simulink model "SF018A_EotProtn"  (R2013b)
settings: Solver=FixedStepDiscrete  SolverMode=SingleTasking  StartTime=0.0  StopTime=0.002  FixedStep=.002  RelTol=1e-3
undefined symbols (not defined in the file): ALLSPDDAMPG_CNT_U08, ALLSPDGAIN_CNT_U08, ARCHGLBPRM_2MILLISEC_SEC_F32, DISTLPFILFRQ_HZ_F32, EOTDAMPGLOLIM_MOTNWTMTR_F32, EOTGAINHILIM_ULS_F32, EotProtnActvRegnBypMaxThd, EotProtnDampgSlew, EotProtnDampgVehSpdTbl, EotProtnDeltaTqThd, EotProtnDftPosn, EotProtnEntrGainVehSpdTbl, EotProtnEntrGainX, EotProtnEntrStLpFilFrq, EotProtnExitDampgY, EotProtnExitStLpFilFrq, EotProtnHwAgGain, EotProtnHwAgMax, EotProtnHwAgMin, EotProtnHwDegDampgX, EotProtnMotSpdIncptSca, EotProtnMotSpdIncptX, EotProtnMotSpdIncptY, EotProtnMotVelGain, EotProtnNormDampgY, EotProtnPosnRampStep, EotProtnRackTrvlLimrAuthyThd, EotProtnRackTrvlLimrAuthyThdLimd, EotProtnRackTrvlLimrEna, EotProtnRackTrvlLimrRng, EotProtnRackTrvlLimrRngLimd, EotProtnRackTrvlLimrVehSpdThd, EotProtnRunEotVelImpctAndSoftEndStop, EotProtnSoftEndStopAuthyThd, EotProtnSoftEndStopEna, EotProtnSoftEndStopVehSpdThd, FIRSTPTDAMPG_CNT_U08, LASTPTGAIN_CNT_U08, SOFTENDSTOPSTDI_CNT_U08, SOFTENDSTOPSTENTR_CNT_U08, SOFTENDSTOPSTEXIT_CNT_U08, SOFTENDSTOPSTNORM_CNT_U08, SYSGLBPRM_MOTTQCMDHILIM_MOTNWTMTR_F32, ZEROMOTTQCMD_MOTNWTMTR_F32
libraries: NxtrAbslt x16, FloatToFixd x14, FixdToFloat x6, Fil x5, NxtrLim x5, simulink x4, NxtrMax x4, LnrIntrpnDyn x3, NxtrSign x2, BilnrIntrpnMplXDyn x2, BilnrIntrpnMplX x1, LnrIntrpn x1
(part 1 of 5)
settings Model: Creator=BZHF94  LastModifiedBy=HZQ8V7
settings DataIOCC: LimitDataPoints=off  SaveFormat=Structure  ReturnWorkspaceOutputs=on
settings OptimizationCC: BlockReduction=off  InlineParams=on  ZeroExternalMemoryAtStartup=off  ZeroInternalMemoryAtStartup=off  OptimizeModelRefInitCode=on  LifeSpan=1
settings DebuggingCC: SignalInfNanChecking=error  SignalRangeChecking=warning  UnderspecifiedInitializationDetection=Simplified  SolverPrmCheckMsg=error  InheritedTsInSrcMsg=error  DiscreteInheritContinuousMsg=error  MultiTaskDSMMsg=none  SingleTaskRateTransMsg=error  TasksWithSamePriorityMsg=error  SigSpecEnsureSampleTimeMsg=error  CheckMatrixSingularityMsg=error  IntegerOverflowMsg=none  ParameterOverflowMsg=none  ParameterUnderflowMsg=error  ParameterPrecisionLossMsg=error  ParameterTunabilityLossMsg=error  FixptConstUnderflowMsg=warning  FixptConstOverflowMsg=warning  VectorMatrixConversionMsg=error  SignalLabelMismatchMsg=error  UnconnectedInputMsg=error  UnconnectedOutputMsg=error  UnconnectedLineMsg=error  SFcnCompatibilityMsg=error  UniqueDataStoreMsg=warning  BusObjectLabelMismatch=error  RootOutportRequireBusObject=error  AssertControl=DisableAll  ModelReferenceIOMsg=error  ModelReferenceVersionMismatchMessage=warning  ModelReferenceIOMismatchMessage=error  ModelReferenceCSMismatchMessage=warning  ModelReferenceDataLoggingMessage=error  StateNameClashWarn=warning  StrictBusMsg=ErrorOnBusTreatedAsVector  NonBusSignalsTreatedAsBus=error  SFUnexpectedBacktrackingDiag=error  SFInvalidInputDataAccessInChartInitDiag=error  SFNoUnconditionalDefaultTransitionDiag=error  SFTransitionOutsideNaturalParentDiag=error  SFUnconditionalTransitionShadowingDiag=error  SFUndirectedBroadcastEventsDiag=error
settings ModelReferenceCC: ModelReferenceNumInstancesAllowed=Single
settings RTWCC: SystemTargetFile=autosar.tlc  GenCodeOnly=on  TemplateMakefile=ert_default_tmf  Description=AUTOSAR  GenerateReport=on  ProcessScript=autosar_make_rtw_hook  LaunchReport=on
settings CodeAppCC: GenerateComments=off  IgnoreCustomStorageClasses=off  CustomSymbolStrType=$N$R$M  CustomSymbolStrBlkIO=$N$M  SimulinkBlockComments=off
settings STFCustomTargetCC: ParMdlRefBuildCompliant=on  CompOptLevelCompliant=on  IncludeMdlTerminateFcn=off  CombineOutputUpdateFcns=on  SuppressErrorStatus=on  ERTFirstTimeCompliant=on  ERTCustomFileBanners=on  SupportNonFinite=off  SupportComplex=off  SupportContinuousTime=off  SupportNonInlinedSFcns=off  MATLABClassNameForMDSCustomization=Simulink.SoftwareTarget.ERTCustomization  AutosarCompliant=on  GRTInterface=off  SystemTargetFile=autosar.tlc
settings ERTTargetCC: CodeReplacementLibrary=ANSI_C  ConcurrentExecutionCompliant=off  IncludeMdlTerminateFcn=off  SuppressErrorStatus=on  SupportNonFinite=off  SupportComplex=off  ModelStepFunctionPrototypeControlCompliant=off  CPPClassGenCompliant=off  AutosarCompliant=on  InlinedParameterPlacement=NonHierarchical  ERTCustomFileTemplate=example_file_process.tlc  EnableUserReplacementTypes=on

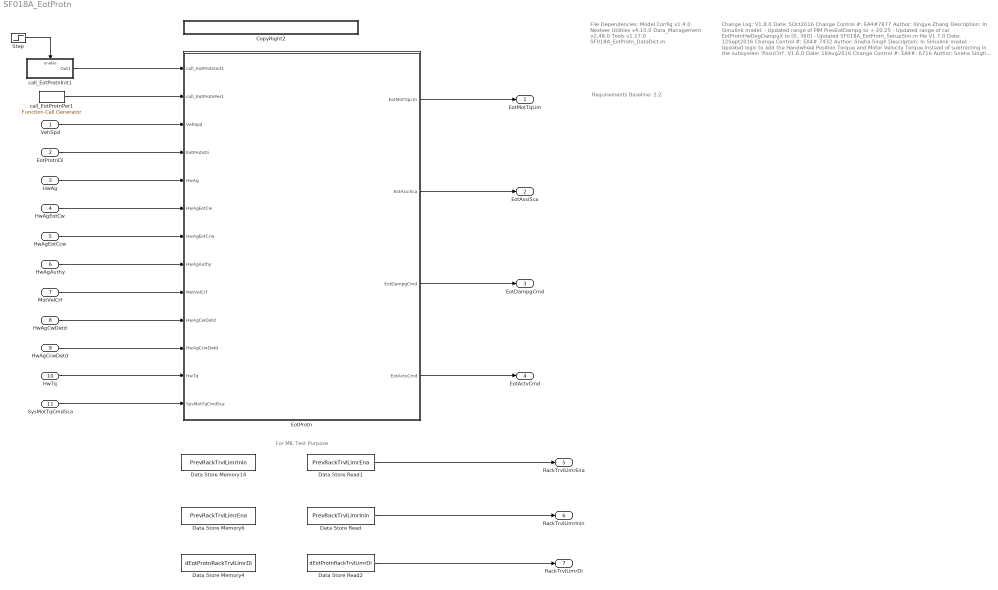
== system SF018A_EotProtn ==
  note: For MIL Test Purpose
  note: File Dependencies:
      |
      | Model Config v1.4.0
      | Nexteer Utilities v4.10.0
      | Data_Management v2.48.0
      | Tools v1.17.0
      | SF018A_EotProtn_DataDict.m
  note: Requirements Baseline: 2.2
  note: Change Log:
      |
      | V1.8.0
      | Date: 5Oct2016
      | Change Control #: EA4#7877
      | Author: Xingye Zhang
      | Description:
      | In Simulink model:
      | - Updated range of PIM PrevEotDampg to +-20.25
      | - Updated range of cal EotProtnHwDegDampgX to [0, 360]
      | - Updated  SF018A_EotProtn_SetupSim.m file
      |
      | V1.7.0
      | Date: 12Sept2016
      | Change Control #: EA4# 7432
      | Author: Sneha Singh
      | Description:
      | In Simulink model:
      | - Updated logic to add the Handwheel Position Torque and Motor Velocity
      | Torque instead of subtracting in the subsystem 'PosnCtrl'.
      |
      | V1.6.0
      | Date: 18Aug2016
      | Change Control #: EA4#: 6716
      | Author: Sneha Singh
      | Description:
      | In DataDictionary:
      | - Updated the filter gain and state variable range.
      | - Updated graphlink for 'EotProtnEntrGainY'.
      | In Simulink model:
      | - Initial values for filter data store blocks updated.
      | - Execution order of 'PrevSoftEndStopSt' updated to read before write.
      | - Deleted AND and NOT blocks from the subsystem 'RackTrvlLimrInin'.
      |
      | V1.5.0
      | Date: 12Jun2016
      | Change Control #: EA4#: 6120
      | Author: Harsh Karve
      | Description
      | In DataDictionary: Added EotProtnRackTrvlLimrAuthyThdLimd
      | 	and EotProtnRackTrvlLimrRngLimd
      | In Simulink model: Added logic to select between
      | 	EotProtnRackTrvlLimrRngLimd and EotProtnRackTrvlLimrRng
      | 	based on EotProtnRackTrvlLimrAuthyThd
      | 	and EotProtnRackTrvlLimrAuthyThdLimd
      |
      | V1.4.0
      | Date: 12Jan2016
      | Change Control #: EA4#3273
      | Author: Sudeep Shankar
      | Description:
      | In DataDictionary, EotProtnRackTrvlLimrEna.EngVal default changed
      | from
      | 1 to 0 to maintain consistency with SF-11
      |
      | V1.3.0
      | Date: 05Oct2015
      | Change Control #: EA4#1019
      | Author: Fei Yuan
      | Description:
      | - Minor values changes on the calibrations:
      |       EotProtnDampgVehSpdTbl
      | 	 EotProtnDftPosn
      | 	 EotProtnEntrGainY
      | 	 EotProtnHwDegDampgX
      | 	 EotProtnMotSpdIncptX
      | 	 EotProtnMotSpdIncptY
      | 	 EotProtnExitDampgY
      |  	 EotProtnNormDampgY
      |  	 EotProtnRackTrvlLimrRng
      |  	 EotProtnRackTrvlLimrVehSpdThd
      |  	 EotProtnSoftEndStopAuthyThd
      | - Unit changes from 'Uls' to 'Cnt' on the constants:
      | 	 ALLSPDDAMPG_CNT_U08
      | 	 ALLSPDGAIN_CNT_U08
      | 	 FIRSTPTDAMPG_CNT_U08
      | 	 LASTPTGAIN_CNT_U08
      |
      |
      | V1.2.0
      | Date: 01Oct2015
      | Change Control #: EA4#1019
      | Author: Fei Yuan
      | Description:
      | - EotAssiSca.WrittenIn is added.
      | - PrevHwTqLpFil is changed to HwTqLpFil.
      | - PrevEotAssiScaLpFil is changed to EotAssiScaLpFil.
      | - LASTROWGAIN_ULS_F32 is changed to LASTPTGAIN_ULS_U08.
      | - FIRSTROWDAMPG_ULS_F32 is changed to FIRSTPTDAMPG_ULS_U08.
      | - ALLCOLGAIN_ULS_F32 is changed to ALLSPDGAIN_ULS_U08.
      | - ALLCOLDAMPG_ULS_U08 is changed to ALLSPDDAMPG_ULS_U08.
      |
      |
      | V 1.1.0
      | Date: 28Sep2015
      | Change Control #: EA4#1019
      | Author: Fei Yuan
      | Description:
      | - Deleting unneeded imported calibration
      | in the Data Dictionary
      |
      |
      | V 1.0.0
      | Date: 15Sep2015
      | Change Control #: EA4#1019
      | Author: Fei Yuan
      | Description:
      | - Initial Release Based on EA3 V 1.0.0
  VehSpd : Inport  RequirementInfo={} %GIDa_f2493df3_3560_4e8c_9ac3_cc4ada172b3a
  EotProtnDi : Inport  RequirementInfo={} %GIDa_9947c430_a5d7_4588_95dd_03f461632271  Port=2
  HwAg : Inport  RequirementInfo={} %GIDa_2659bb7a_c59e_415b_8b99_460c1be3fe4a  Port=3
  HwAgEotCw : Inport  RequirementInfo={} %GIDa_b8d4db66_b9a1_483c_9e62_5724d2f818de  Port=4
  HwAgEotCcw : Inport  RequirementInfo={} %GIDa_ddb9e909_8804_448b_851e_077ef608e27a  Port=5
  HwAgAuthy : Inport  RequirementInfo={} %GIDa_073559df_e8e0_40c2_83ff_8c97959cf4b7  Port=6
  MotVelCrf : Inport  RequirementInfo={} %GIDa_06a07364_6048_4403_8ccd_af20484cf926  Port=7
  HwAgCwDetd : Inport  RequirementInfo={} %GIDa_c86b3aa5_494e_4d5c_8b58_596cd01b1b79  Port=8
  HwAgCcwDetd : Inport  RequirementInfo={} %GIDa_6f73f07d_03be_4ab3_ac9e_f6331c6d0b68  Port=9
  HwTq : Inport  RequirementInfo={} %GIDa_3422e606_a4dc_43df_b15d_a957c57f1483  Port=10
  SysMotTqCmdSca : Inport  RequirementInfo={} %GIDa_5f2ee495_d7fd_4bfd_8356_7328f9a76091  Port=11
  CopyRight2 : Subsystem  Description=|  mask(Copyright Information){none=on}
      | Copyright info block.                                               
      |                                                                     
      | Place copyright information at the top of every subsystem in design.
      mask prompts: none "No parameters"
      mask help: Place copyright information at the top of every subsystem in design.
      mask Display:
      | NxtrConf = 'Nexteer Confidential';
      | 
      | sys = bdroot; %handle for the current model ("system")
      | first = get_param(sys,'Created');
      | if(isempty(first))
      |     first = datestr(now,'yyyy');
      | else
      |     first = first(end-3:end);  %year is last four digits
      | end
      | 
      | last = get_param(sys,'LastModifiedDate');
      | if isempty(last)
      |     last = datestr(now,'yyyy');
      | else
      |     last = last(end-3:end);
      | end
      | 
      | if strcmp(first,last)
      |     fprintf('%s -- Copyright %s Nexteer',NxtrConf,first)
      | else
      |     fprintf('%s -- %s%s- %s Nexteer',NxtrConf,char(169),first,last)
      | end
  Data Store Memory14 : DataStoreMemory  DataStoreName=PrevRackTrvlLimrInin  StateMustResolveToSignalObject=on
  Data Store Memory4 : DataStoreMemory  DataStoreName=dEotProtnRackTrvlLimrDi  StateMustResolveToSignalObject=on
  Data Store Memory6 : DataStoreMemory  DataStoreName=PrevRackTrvlLimrEna  StateMustResolveToSignalObject=on
  Data Store Read : DataStoreRead  DataStoreName=PrevRackTrvlLimrInin  SampleTime=0.002
  Data Store Read1 : DataStoreRead  DataStoreName=PrevRackTrvlLimrEna  SampleTime=0.002
  Data Store Read2 : DataStoreRead  DataStoreName=dEotProtnRackTrvlLimrDi  SampleTime=0.002
  EotProtn : Subsystem
  Step : Step  Time=.001  Before=1  After=0  SampleTime=0
  call_EotProtnInit1 : Subsystem  TreatAsAtomicUnit=on
  call_EotProtnPer1 : simulink/Ports & Subsystems/Function-Call Generator  RequirementInfo={} %GIDa_6f959799_a3aa_4853_a8c2_1b349d8a0077  sample_time=0.002  numberOfIterations=1
  EotMotTqLim : Outport
  EotAssiSca : Outport  Port=2
  EotDampgCmd : Outport  Port=3
  EotActvCmd : Outport  Port=4
  RackTrvlLimrEna : Outport  Port=5
  RackTrvlLimrInin : Outport  Port=6
  RackTrvlLimrDi : Outport  Port=7
  wires:
  EotProtn/1(EotMotTqLim) -> EotMotTqLim/1
  EotProtn/4(EotActvCmd) -> EotActvCmd/1
  EotProtn/3(EotDampgCmd) -> EotDampgCmd/1
  EotProtn/2(EotAssiSca) -> EotAssiSca/1
  Data Store Read/1 -> RackTrvlLimrInin/1
  Data Store Read1/1 -> RackTrvlLimrEna/1
  Data Store Read2/1 -> RackTrvlLimrDi/1
  Step/1 -> call_EotProtnInit1/Enable
  call_EotProtnPer1/1 -> EotProtn/2(call_EotProtnPer1)
  call_EotProtnInit1/1(Out1) -> EotProtn/1(call_EotProtnInit1)
  VehSpd/1 -> EotProtn/3(VehSpd)
  EotProtnDi/1 -> EotProtn/4(EotProtnDi)
  HwAg/1 -> EotProtn/5(HwAg)
  HwAgEotCw/1 -> EotProtn/6(HwAgEotCw)
  HwAgEotCcw/1 -> EotProtn/7(HwAgEotCcw)
  HwAgAuthy/1 -> EotProtn/8(HwAgAuthy)
  MotVelCrf/1 -> EotProtn/9(MotVelCrf)
  HwAgCwDetd/1 -> EotProtn/10(HwAgCwDetd)
  HwAgCcwDetd/1 -> EotProtn/11(HwAgCcwDetd)
  HwTq/1 -> EotProtn/12(HwTq)
  SysMotTqCmdSca/1 -> EotProtn/13(SysMotTqCmdSca)

== system SF018A_EotProtn/CopyRight2 ==

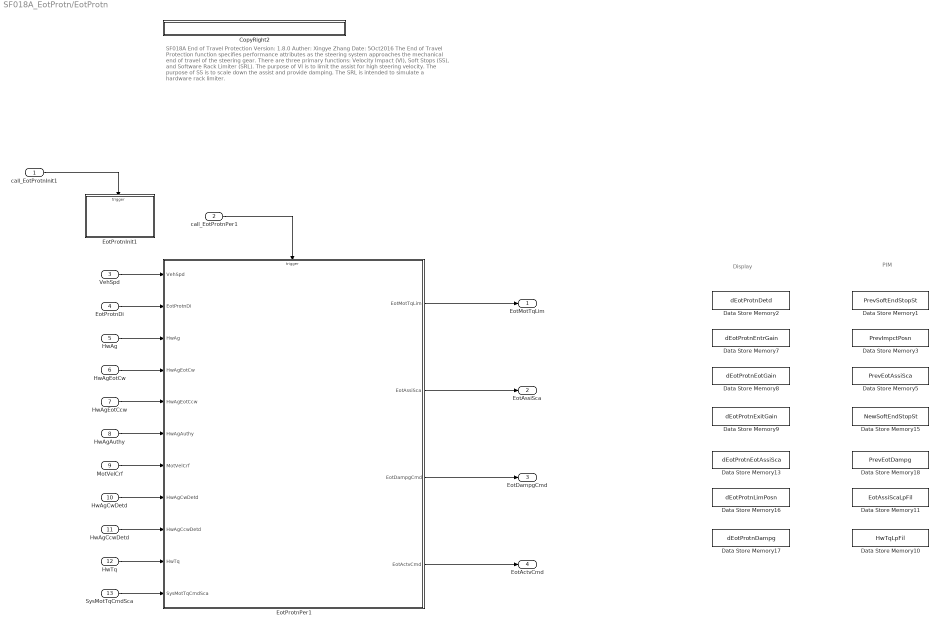
== system SF018A_EotProtn/EotProtn ==
  note: PIM
  note: Display
  note: SF018A End of Travel Protection
      | Version: 1.8.0  Auther: Xingye Zhang       Date: 5Oct2016
      |
      | The End of Travel Protection function specifies performance attributes as the steering system approaches the mechanical end of travel
      | of the steering gear. There are three primary functions: Velocity Impact (VI), Soft Stops (SS), and Software Rack Limiter (SRL).
      |
      | The purpose of VI is to limit the assist for high steering velocity. The purpose of SS is to scale down the assist and provide damping. The
      | SRL is intended to simulate a hardware rack limiter.
  call_EotProtnInit1 : Inport
  call_EotProtnPer1 : Inport  Port=2
  VehSpd : Inport  RequirementInfo={'linktype_rmi_doors' '0000ba56 (/E-STEER Core/SubSystem Specifications/Application Functions/SF018A End-of-Travel Actuator Management- EOT Impact and Soft Stops)' '#SF018A_39' 'true' 'REQ: SF018A_39' '' } %GIDa_a78556f8_403e_4502_952b_ada00a94acb5  Port=3
  EotProtnDi : Inport  RequirementInfo={'linktype_rmi_doors' '0000ba56 (/E-STEER Core/SubSystem Specifications/Application Functions/SF018A End-of-Travel Actuator Management- EOT Impact and Soft Stops)' '#SF018A_40' 'true' 'REQ: SF018A_40' '' } %GIDa_b64a771e_65c5_4ece_b91a_db7d931b086f  Port=4
  HwAg : Inport  RequirementInfo={'linktype_rmi_doors' '0000ba56 (/E-STEER Core/SubSystem Specifications/Application Functions/SF018A End-of-Travel Actuator Management- EOT Impact and Soft Stops)' '#SF018A_41' 'true' 'REQ: SF018A_41' '' } %GIDa_eecdc59f_15cc_4f2b_ad72_cb34d73e8cb8  Port=5
  HwAgEotCw : Inport  RequirementInfo={'linktype_rmi_doors' '0000ba56 (/E-STEER Core/SubSystem Specifications/Application Functions/SF018A End-of-Travel Actuator Management- EOT Impact and Soft Stops)' '#SF018A_81' 'true' 'REQ: SF018A_81' '' } %GIDa_23f8dc21_a30b_406d_bb74_847676667852  Port=6
  HwAgEotCcw : Inport  RequirementInfo={'linktype_rmi_doors' '0000ba56 (/E-STEER Core/SubSystem Specifications/Application Functions/SF018A End-of-Travel Actuator Management- EOT Impact and Soft Stops)' '#SF018A_82' 'true' 'REQ: SF018A_82' '' } %GIDa_6c945122_f602_4615_8a0d_9b6a5b36fdce  Port=7
  HwAgAuthy : Inport  RequirementInfo={'linktype_rmi_doors' '0000ba56 (/E-STEER Core/SubSystem Specifications/Application Functions/SF018A End-of-Travel Actuator Management- EOT Impact and Soft Stops)' '#SF018A_42' 'true' 'REQ: SF018A_42' '' } %GIDa_097a9b08_a5d5_46d9_827a_8d91469ca1ea  Port=8
  MotVelCrf : Inport  RequirementInfo={'linktype_rmi_doors' '0000ba56 (/E-STEER Core/SubSystem Specifications/Application Functions/SF018A End-of-Travel Actuator Management- EOT Impact and Soft Stops)' '#SF018A_38' 'true' 'REQ: SF018A_38' '' } %GIDa_1a8588a9_3d2e_48f3_a762_af26475c6c5c  Port=9
  HwAgCwDetd : Inport  RequirementInfo={'linktype_rmi_doors' '0000ba56 (/E-STEER Core/SubSystem Specifications/Application Functions/SF018A End-of-Travel Actuator Management- EOT Impact and Soft Stops)' '#SF018A_43' 'true' 'REQ: SF018A_43' '' } %GIDa_b5da2d0c_99ae_4332_b60f_c5663cccbdf6  Port=10
  HwAgCcwDetd : Inport  RequirementInfo={'linktype_rmi_doors' '0000ba56 (/E-STEER Core/SubSystem Specifications/Application Functions/SF018A End-of-Travel Actuator Management- EOT Impact and Soft Stops)' '#SF018A_80' 'true' 'REQ: SF018A_80' '' } %GIDa_337a4959_1d61_4717_9ff7_4d7f36a2ed66  Port=11
  HwTq : Inport  RequirementInfo={'linktype_rmi_doors' '0000ba56 (/E-STEER Core/SubSystem Specifications/Application Functions/SF018A End-of-Travel Actuator Management- EOT Impact and Soft Stops)' '#SF018A_18' 'true' 'REQ: SF018A_18' '' } %GIDa_c0387548_ba78_41a1_af32_a62cdacc5f34  Port=12
  SysMotTqCmdSca : Inport  RequirementInfo={'linktype_rmi_doors' '0000ba56 (/E-STEER Core/SubSystem Specifications/Application Functions/SF018A End-of-Travel Actuator Management- EOT Impact and Soft Stops)' '#SF018A_156' 'true' 'REQ: SF018A_156' '' } %GIDa_0ae76b0a_9341_4fdf_8ebd_214537950b15  Port=13
  CopyRight2 : Subsystem  Description=|  mask(Copyright Information){none=on}
      | Copyright info block.                                               
      |                                                                     
      | Place copyright information at the top of every subsystem in design.
      mask prompts: none "No parameters"
      mask help: Place copyright information at the top of every subsystem in design.
      mask Display:
      | NxtrConf = 'Nexteer Confidential';
      | 
      | sys = bdroot; %handle for the current model ("system")
      | first = get_param(sys,'Created');
      | if(isempty(first))
      |     first = datestr(now,'yyyy');
      | else
      |     first = first(end-3:end);  %year is last four digits
      | end
      | 
      | last = get_param(sys,'LastModifiedDate');
      | if isempty(last)
      |     last = datestr(now,'yyyy');
      | else
      |     last = last(end-3:end);
      | end
      | 
      | if strcmp(first,last)
      |     fprintf('%s -- Copyright %s Nexteer',NxtrConf,first)
      | else
      |     fprintf('%s -- %s%s- %s Nexteer',NxtrConf,char(169),first,last)
      | end
  Data Store Memory1 : DataStoreMemory  DataStoreName=PrevSoftEndStopSt  StateMustResolveToSignalObject=on
  Data Store Memory10 : DataStoreMemory  DataStoreName=HwTqLpFil  InitialValue=[]  OutDataTypeStr=Bus: FilLpRec1  StateMustResolveToSignalObject=on
  Data Store Memory11 : DataStoreMemory  DataStoreName=EotAssiScaLpFil  InitialValue=[]  OutDataTypeStr=Bus: FilLpRec1  StateMustResolveToSignalObject=on
  Data Store Memory13 : DataStoreMemory  DataStoreName=dEotProtnEotAssiSca  ReadBeforeWriteMsg=warning  WriteAfterWriteMsg=warning  WriteAfterReadMsg=warning  StateMustResolveToSignalObject=on
  Data Store Memory15 : DataStoreMemory  DataStoreName=NewSoftEndStopSt  StateMustResolveToSignalObject=on
  Data Store Memory16 : DataStoreMemory  DataStoreName=dEotProtnLimPosn  ReadBeforeWriteMsg=warning  WriteAfterWriteMsg=warning  WriteAfterReadMsg=warning  StateMustResolveToSignalObject=on
  Data Store Memory17 : DataStoreMemory  DataStoreName=dEotProtnDampg  ReadBeforeWriteMsg=warning  WriteAfterWriteMsg=warning  WriteAfterReadMsg=warning  StateMustResolveToSignalObject=on
  Data Store Memory18 : DataStoreMemory  DataStoreName=PrevEotDampg  StateMustResolveToSignalObject=on
  Data Store Memory2 : DataStoreMemory  DataStoreName=dEotProtnDetd  ReadBeforeWriteMsg=warning  WriteAfterWriteMsg=warning  WriteAfterReadMsg=warning  StateMustResolveToSignalObject=on
  Data Store Memory3 : DataStoreMemory  DataStoreName=PrevImpctPosn  StateMustResolveToSignalObject=on
  Data Store Memory5 : DataStoreMemory  DataStoreName=PrevEotAssiSca  StateMustResolveToSignalObject=on
  Data Store Memory7 : DataStoreMemory  DataStoreName=dEotProtnEntrGain  ReadBeforeWriteMsg=warning  WriteAfterWriteMsg=warning  WriteAfterReadMsg=warning  StateMustResolveToSignalObject=on
  Data Store Memory8 : DataStoreMemory  DataStoreName=dEotProtnEotGain  ReadBeforeWriteMsg=warning  WriteAfterWriteMsg=warning  WriteAfterReadMsg=warning  StateMustResolveToSignalObject=on
  Data Store Memory9 : DataStoreMemory  DataStoreName=dEotProtnExitGain  ReadBeforeWriteMsg=warning  WriteAfterWriteMsg=warning  WriteAfterReadMsg=warning  StateMustResolveToSignalObject=on
  EotProtnInit1 : Subsystem
  EotProtnPer1 : Subsystem
  EotMotTqLim : Outport  RequirementInfo={'linktype_rmi_doors' '0000ba56 (/E-STEER Core/SubSystem Specifications/Application Functions/SF018A End-of-Travel Actuator Management- EOT Impact and Soft Stops)' '#SF018A_20' 'true' 'REQ: SF018A_20' '' } %GIDa_69ec1092_67bc_4a3b_9f2e_0b0963ae28ca
  EotAssiSca : Outport  RequirementInfo={'linktype_rmi_doors' '0000ba56 (/E-STEER Core/SubSystem Specifications/Application Functions/SF018A End-of-Travel Actuator Management- EOT Impact and Soft Stops)' '#SF018A_44' 'true' 'REQ: SF018A_44' '' } %GIDa_1d9dfd8d_4c50_4570_b0ff_14c703a96e1d  Port=2
  EotDampgCmd : Outport  RequirementInfo={'linktype_rmi_doors' '0000ba56 (/E-STEER Core/SubSystem Specifications/Application Functions/SF018A End-of-Travel Actuator Management- EOT Impact and Soft Stops)' '#SF018A_45' 'true' 'REQ: SF018A_45' '' } %GIDa_758b54e5_2560_4187_be88_11d99f480d4d  Port=3
  EotActvCmd : Outport  RequirementInfo={'linktype_rmi_doors' '0000ba56 (/E-STEER Core/SubSystem Specifications/Application Functions/SF018A End-of-Travel Actuator Management- EOT Impact and Soft Stops)' '#SF018A_83' 'true' 'REQ: SF018A_83' '' } %GIDa_02248581_82c0_43b2_970c_42c45dcb5430  Port=4
  wires:
  SysMotTqCmdSca/1 -> EotProtnPer1/11(SysMotTqCmdSca)
  call_EotProtnInit1/1 -> EotProtnInit1/Trigger
  call_EotProtnPer1/1 -> EotProtnPer1/Trigger
  HwAg/1 -> EotProtnPer1/3(HwAg)
  HwAgCcwDetd/1 -> EotProtnPer1/9(HwAgCcwDetd)
  EotProtnPer1/3(EotDampgCmd) -> EotDampgCmd/1
  HwAgEotCcw/1 -> EotProtnPer1/5(HwAgEotCcw)
  VehSpd/1 -> EotProtnPer1/1(VehSpd)
  HwAgEotCw/1 -> EotProtnPer1/4(HwAgEotCw)
  EotProtnDi/1 -> EotProtnPer1/2(EotProtnDi)
  HwAgCwDetd/1 -> EotProtnPer1/8(HwAgCwDetd)
  EotProtnPer1/2(EotAssiSca) -> EotAssiSca/1
  HwTq/1 -> EotProtnPer1/10(HwTq)
  MotVelCrf/1 -> EotProtnPer1/7(MotVelCrf)
  EotProtnPer1/1(EotMotTqLim) -> EotMotTqLim/1
  EotProtnPer1/4(EotActvCmd) -> EotActvCmd/1
  HwAgAuthy/1 -> EotProtnPer1/6(HwAgAuthy)

== system SF018A_EotProtn/call_EotProtnInit1 ==
  Enable : EnablePort
  CopyRight2 : Subsystem  Description=|  mask(Copyright Information){none=on}
      | Copyright info block.                                               
      |                                                                     
      | Place copyright information at the top of every subsystem in design.
      mask prompts: none "No parameters"
      mask help: Place copyright information at the top of every subsystem in design.
      mask Display:
      | NxtrConf = 'Nexteer Confidential';
      | 
      | sys = bdroot; %handle for the current model ("system")
      | first = get_param(sys,'Created');
      | if(isempty(first))
      |     first = datestr(now,'yyyy');
      | else
      |     first = first(end-3:end);  %year is last four digits
      | end
      | 
      | last = get_param(sys,'LastModifiedDate');
      | if isempty(last)
      |     last = datestr(now,'yyyy');
      | else
      |     last = last(end-3:end);
      | end
      | 
      | if strcmp(first,last)
      |     fprintf('%s -- Copyright %s Nexteer',NxtrConf,first)
      | else
      |     fprintf('%s -- %s%s- %s Nexteer',NxtrConf,char(169),first,last)
      | end
  Function_Call_Generator : simulink/Ports & Subsystems/Function-Call Generator  sample_time=0  numberOfIterations=1
  Out1 : Outport
  wires:
  Function_Call_Generator/1 -> Out1/1

== system SF018A_EotProtn/EotProtn/CopyRight2 ==

== system SF018A_EotProtn/EotProtn/EotProtnInit1 ==
  function : TriggerPort  TriggerType=function-call
  CopyRight2 : Subsystem  Description=|  mask(Copyright Information){none=on}
      | Copyright info block.                                               
      |                                                                     
      | Place copyright information at the top of every subsystem in design.
      mask prompts: none "No parameters"
      mask help: Place copyright information at the top of every subsystem in design.
      mask Display:
      | NxtrConf = 'Nexteer Confidential';
      | 
      | sys = bdroot; %handle for the current model ("system")
      | first = get_param(sys,'Created');
      | if(isempty(first))
      |     first = datestr(now,'yyyy');
      | else
      |     first = first(end-3:end);  %year is last four digits
      | end
      | 
      | last = get_param(sys,'LastModifiedDate');
      | if isempty(last)
      |     last = datestr(now,'yyyy');
      | else
      |     last = last(end-3:end);
      | end
      | 
      | if strcmp(first,last)
      |     fprintf('%s -- Copyright %s Nexteer',NxtrConf,first)
      | else
      |     fprintf('%s -- %s%s- %s Nexteer',NxtrConf,char(169),first,last)
      | end
  EotAssiScaLpFil : Fil/FilLpInit  RequirementInfo={'linktype_rmi_doors' '0000ba56 (/E-STEER Core/SubSystem Specifications/Application Functions/SF018A End-of-Travel Actuator Management- EOT Impact and Soft Stops)' '#SF018A_111' 'true' 'REQ: SF018A_111' '' } %GIDa_a2f99997_2c39_4020_9932_83fabe8f4401  Ic=0  Ts=ARCHGLBPRM_2MILLISEC_SEC_F32  Freq=DISTLPFILFRQ_HZ_F32  StVar=EotAssiScaLpFil
  HwTqLpFil : Fil/FilLpInit  Ic=0  Ts=ARCHGLBPRM_2MILLISEC_SEC_F32  Freq=EotProtnHwTqLpFilFrq  StVar=HwTqLpFil

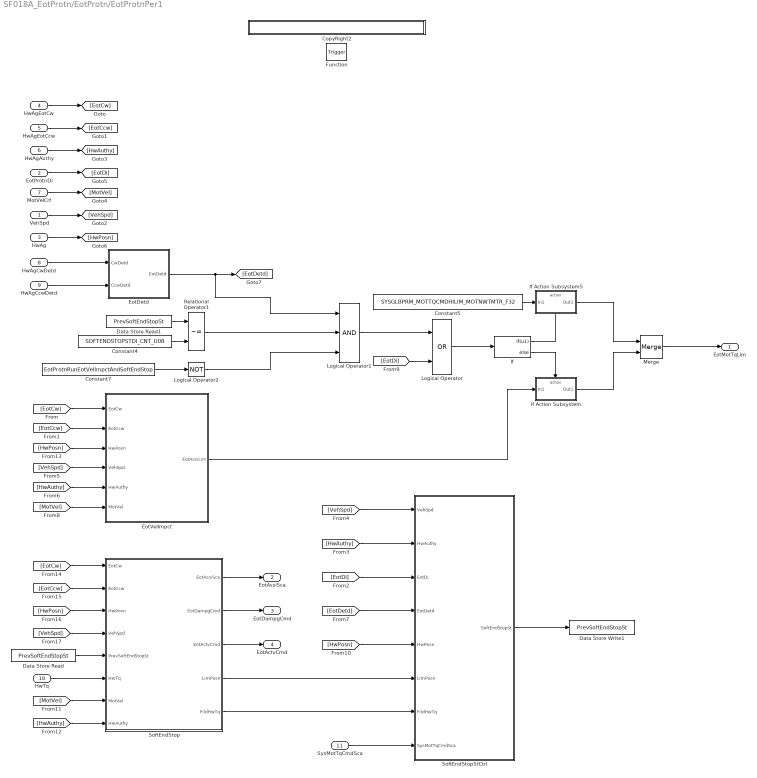
== system SF018A_EotProtn/EotProtn/EotProtnPer1 ==
  VehSpd : Inport
  EotProtnDi : Inport  Port=2
  HwAg : Inport  Port=3
  HwAgEotCw : Inport  Port=4
  HwAgEotCcw : Inport  Port=5
  HwAgAuthy : Inport  Port=6
  MotVelCrf : Inport  Port=7
  HwAgCwDetd : Inport  Port=8
  HwAgCcwDetd : Inport  Port=9
  HwTq : Inport  Port=10
  SysMotTqCmdSca : Inport  Port=11
  Function : TriggerPort  TriggerType=function-call  PortDimensions=1
  Constant4 : Constant  RequirementInfo={'linktype_rmi_doors' '0000ba56 (/E-STEER Core/SubSystem Specifications/Application Functions/SF018A End-of-Travel Actuator Management- EOT Impact and Soft Stops)' '#SF018A_101' 'true' 'REQ: SF018A_101' '' ; 'linktype_rmi_doors' '0000ba56 (/E-STEER Core/SubSystem Specifications/Application Functions/SF018A End-of-Travel Actuator Management- EOT Impact and Soft Stops)' '#SF018A_102' 'true' 'REQ: SF018A_102' '' } %GIDa_61ceba65_7d2a_487b_92a1_1928ed0fb012  Value=SOFTENDSTOPSTDI_CNT_U08
  Constant5 : Constant  RequirementInfo={'linktype_rmi_doors' '0000ba56 (/E-STEER Core/SubSystem Specifications/Application Functions/SF018A End-of-Travel Actuator Management- EOT Impact and Soft Stops)' '#SF018A_98' 'true' 'REQ: SF018A_98' '' } %GIDa_90b24707_b12d_4a90_a810_c09b59997368  Value=SYSGLBPRM_MOTTQCMDHILIM_MOTNWTMTR_F32
  Constant7 : Constant  RequirementInfo={'linktype_rmi_doors' '0000ba56 (/E-STEER Core/SubSystem Specifications/Application Functions/SF018A End-of-Travel Actuator Management- EOT Impact and Soft Stops)' '#SF018A_101' 'true' 'REQ: SF018A_101' '' ; 'linktype_rmi_doors' '0000ba56 (/E-STEER Core/SubSystem Specifications/Application Functions/SF018A End-of-Travel Actuator Management- EOT Impact and Soft Stops)' '#SF018A_102' 'true' 'REQ: SF018A_102' '' } %GIDa_55945f38_9a94_4e4b_989e_25efa663017a  Value=EotProtnRunEotVelImpctAndSoftEndStop
  CopyRight2 : Subsystem  Description=|  mask(Copyright Information){none=on}
      | Copyright info block.                                               
      |                                                                     
      | Place copyright information at the top of every subsystem in design.
      mask prompts: none "No parameters"
      mask help: Place copyright information at the top of every subsystem in design.
      mask Display:
      | NxtrConf = 'Nexteer Confidential';
      | 
      | sys = bdroot; %handle for the current model ("system")
      | first = get_param(sys,'Created');
      | if(isempty(first))
      |     first = datestr(now,'yyyy');
      | else
      |     first = first(end-3:end);  %year is last four digits
      | end
      | 
      | last = get_param(sys,'LastModifiedDate');
      | if isempty(last)
      |     last = datestr(now,'yyyy');
      | else
      |     last = last(end-3:end);
      | end
      | 
      | if strcmp(first,last)
      |     fprintf('%s -- Copyright %s Nexteer',NxtrConf,first)
      | else
      |     fprintf('%s -- %s%s- %s Nexteer',NxtrConf,char(169),first,last)
      | end
  Data Store Read : DataStoreRead  Priority=1  DataStoreName=PrevSoftEndStopSt
      settings: AttributesFormatString=Priority:%<Priority>
  Data Store Read1 : DataStoreRead  RequirementInfo={'linktype_rmi_doors' '0000ba56 (/E-STEER Core/SubSystem Specifications/Application Functions/SF018A End-of-Travel Actuator Management- EOT Impact and Soft Stops)' '#SF018A_101' 'true' 'REQ: SF018A_101' '' ; 'linktype_rmi_doors' '0000ba56 (/E-STEER Core/SubSystem Specifications/Application Functions/SF018A End-of-Travel Actuator Management- EOT Impact and Soft Stops)' '#SF018A_102' 'true' 'REQ: SF018A_102' '' } %GIDa_fe59ddd6_b037_49ff_8cce_f0538ffbce85  Priority=1  DataStoreName=PrevSoftEndStopSt
      settings: AttributesFormatString=Priority:%<Priority>
  Data Store Write1 : DataStoreWrite  Priority=2  DataStoreName=PrevSoftEndStopSt
      settings: AttributesFormatString=Priority:%<Priority>
  EotDetd : Subsystem  RequirementInfo={'linktype_rmi_doors' '0000ba56 (/E-STEER Core/SubSystem Specifications/Application Functions/SF018A End-of-Travel Actuator Management- EOT Impact and Soft Stops)' '#SF018A_102' 'true' 'REQ: SF018A_102' '' ; 'linktype_rmi_doors' '0000ba56 (/E-STEER Core/SubSystem Specifications/Application Functions/SF018A End-of-Travel Actuator Management- EOT Impact and Soft Stops)' '#SF018A_101' 'true' 'REQ: SF018A_101' '' } %GIDa_80696681_6200_4575_abaf_6bc99a1cbedb  TreatAsAtomicUnit=on
  EotVelImpct : Subsystem
      settings: AttributesFormatString=Original End of Travel Impact Routine
  If : If  RequirementInfo={'linktype_rmi_doors' '0000ba56 (/E-STEER Core/SubSystem Specifications/Application Functions/SF018A End-of-Travel Actuator Management- EOT Impact and Soft Stops)' '#SF018A_98' 'true' 'REQ: SF018A_98' '' } %GIDa_0af2b1e4_5307_4cd8_9dde_c7a53b641615  IfExpression=u1
  If Action Subsystem : Subsystem  RequirementInfo={'linktype_rmi_doors' '0000ba56 (/E-STEER Core/SubSystem Specifications/Application Functions/SF018A End-of-Travel Actuator Management- EOT Impact and Soft Stops)' '#SF018A_98' 'true' 'REQ: SF018A_98' '' } %GIDa_9161bff8_7a81_4d99_b146_c5833750b158  TreatAsAtomicUnit=on
  If Action Subsystem5 : Subsystem  RequirementInfo={'linktype_rmi_doors' '0000ba56 (/E-STEER Core/SubSystem Specifications/Application Functions/SF018A End-of-Travel Actuator Management- EOT Impact and Soft Stops)' '#SF018A_98' 'true' 'REQ: SF018A_98' '' } %GIDa_6238493d_2916_4e86_a7f1_4536482b874e  TreatAsAtomicUnit=on
  Logical Operator : Logic  RequirementInfo={'linktype_rmi_doors' '0000ba56 (/E-STEER Core/SubSystem Specifications/Application Functions/SF018A End-of-Travel Actuator Management- EOT Impact and Soft Stops)' '#SF018A_101' 'true' 'REQ: SF018A_101' '' ; 'linktype_rmi_doors' '0000ba56 (/E-STEER Core/SubSystem Specifications/Application Functions/SF018A End-of-Travel Actuator Management- EOT Impact and Soft Stops)' '#SF018A_104' 'true' 'REQ: SF018A_104' '' ; 'linktype_rmi_doors' '0000ba56 (/E-STEER Core/SubSystem Specifications/Application Functions/SF018A End-of-Travel Actuator Management- EOT Impact and Soft Stops)' '#SF018A_102' 'true' 'REQ: SF018A_102' '' ; 'linktype_rmi_doors' '0000ba56 (/E-STEER Core/SubSystem Specifications/Application Functions/SF018A End-of-Travel Actuator Management- EOT Impact and Soft Stops)' '#SF018A_103' 'true' 'REQ: SF018A_103' '' } %GIDa_53250173_a2d5_42a0_8e96_11b163e82ec1  Operator=OR  AllPortsSameDT=off  OutDataTypeStr=boolean
  Logical Operator1 : Logic  RequirementInfo={'linktype_rmi_doors' '0000ba56 (/E-STEER Core/SubSystem Specifications/Application Functions/SF018A End-of-Travel Actuator Management- EOT Impact and Soft Stops)' '#SF018A_101' 'true' 'REQ: SF018A_101' '' ; 'linktype_rmi_doors' '0000ba56 (/E-STEER Core/SubSystem Specifications/Application Functions/SF018A End-of-Travel Actuator Management- EOT Impact and Soft Stops)' '#SF018A_102' 'true' 'REQ: SF018A_102' '' ; 'linktype_rmi_doors' '0000ba56 (/E-STEER Core/SubSystem Specifications/Application Functions/SF018A End-of-Travel Actuator Management- EOT Impact and Soft Stops)' '#SF018A_104' 'true' 'REQ: SF018A_104' '' } %GIDa_cbf4a1f3_742c_4859_9101_f4df2ead0d3f  Inputs=3  AllPortsSameDT=off  OutDataTypeStr=boolean
  Logical Operator2 : Logic  RequirementInfo={'linktype_rmi_doors' '0000ba56 (/E-STEER Core/SubSystem Specifications/Application Functions/SF018A End-of-Travel Actuator Management- EOT Impact and Soft Stops)' '#SF018A_101' 'true' 'REQ: SF018A_101' '' ; 'linktype_rmi_doors' '0000ba56 (/E-STEER Core/SubSystem Specifications/Application Functions/SF018A End-of-Travel Actuator Management- EOT Impact and Soft Stops)' '#SF018A_102' 'true' 'REQ: SF018A_102' '' } %GIDa_8e66e37e_ae4e_4930_9ca8_0803fdd90e09  Operator=NOT  AllPortsSameDT=off  OutDataTypeStr=boolean
  Merge : Merge  RequirementInfo={'linktype_rmi_doors' '0000ba56 (/E-STEER Core/SubSystem Specifications/Application Functions/SF018A End-of-Travel Actuator Management- EOT Impact and Soft Stops)' '#SF018A_98' 'true' 'REQ: SF018A_98' '' } %GIDa_88146030_7d58_4732_8048_ebe090fceeca
  Relational Operator1 : RelationalOperator  RequirementInfo={'linktype_rmi_doors' '0000ba56 (/E-STEER Core/SubSystem Specifications/Application Functions/SF018A End-of-Travel Actuator Management- EOT Impact and Soft Stops)' '#SF018A_101' 'true' 'REQ: SF018A_101' '' ; 'linktype_rmi_doors' '0000ba56 (/E-STEER Core/SubSystem Specifications/Application Functions/SF018A End-of-Travel Actuator Management- EOT Impact and Soft Stops)' '#SF018A_102' 'true' 'REQ: SF018A_102' '' } %GIDa_27a9dc10_b944_427a_8b47_3f76c0679fad  Operator=~=  OutDataTypeStr=boolean
  SoftEndStop : Subsystem
  SoftEndStopStCtrl : Subsystem
      settings: AttributesFormatString=Soft End Stop State Control
  EotMotTqLim : Outport
  EotAssiSca : Outport  Port=2
  EotDampgCmd : Outport  Port=3
  EotActvCmd : Outport  Port=4
  wires:
  Relational Operator1/1 -> Logical Operator1/2
  EotDetd/1(EotDetd) -> [EotDetd], Logical Operator1/1
  Merge/1 -> EotMotTqLim/1
  Constant4/1 -> Relational Operator1/2
  Data Store Read1/1 -> Relational Operator1/1
  SysMotTqCmdSca/1 -> SoftEndStopStCtrl/8(SysMotTqCmdSca)
  SoftEndStopStCtrl/1(SoftEndStopSt) -> Data Store Write1/1
  SoftEndStop/1(EotAssiSca) -> EotAssiSca/1
  Data Store Read/1 -> SoftEndStop/5(PrevSoftEndStopSt)
  [VehSpd] -> SoftEndStop/4(VehSpd)
  [HwPosn] -> SoftEndStop/3(HwPosn)
  [EotCcw] -> SoftEndStop/2(EotCcw)
  [EotCw] -> SoftEndStop/1(EotCw)
  [HwAuthy] -> SoftEndStop/8(HwAuthy)
  [MotVel] -> SoftEndStop/7(MotVel)
  HwTq/1 -> SoftEndStop/6(HwTq)
  SoftEndStop/3(EotActvCmd) -> EotActvCmd/1
  SoftEndStop/2(EotDampgCmd) -> EotDampgCmd/1
  If Action Subsystem/1(Out1) -> Merge/2
  If Action Subsystem5/1(Out1) -> Merge/1
  If/2 -> If Action Subsystem/Action
  If/1 -> If Action Subsystem5/Action
  Logical Operator2/1 -> Logical Operator1/3
  Logical Operator1/1 -> Logical Operator/1
  [EotDi] -> Logical Operator/2
  Logical Operator/1 -> If/1
  Constant7/1 -> Logical Operator2/1
  HwAgCcwDetd/1 -> EotDetd/2(CcwDetd)
  HwAgCwDetd/1 -> EotDetd/1(CwDetd)
  HwAg/1 -> [HwPosn]
  EotProtnDi/1 -> [EotDi]
  HwAgAuthy/1 -> [HwAuthy]
  MotVelCrf/1 -> [MotVel]
  VehSpd/1 -> [VehSpd]
  HwAgEotCcw/1 -> [EotCcw]
  HwAgEotCw/1 -> [EotCw]
  [VehSpd] -> EotVelImpct/4(VehSpd)
  [MotVel] -> EotVelImpct/6(MotVel)
  [EotCw] -> EotVelImpct/1(EotCw)
  [HwAuthy] -> EotVelImpct/5(HwAuthy)
  [EotCcw] -> EotVelImpct/2(EotCcw)
  [HwPosn] -> EotVelImpct/3(HwPosn)
  EotVelImpct/1(EotAssiLim) -> If Action Subsystem/1(In1)
  SoftEndStop/5(FildHwTq) -> SoftEndStopStCtrl/7(FildHwTq)
  SoftEndStop/4(LimPosn) -> SoftEndStopStCtrl/6(LimPosn)
  [HwPosn] -> SoftEndStopStCtrl/5(HwPosn)
  [EotDetd] -> SoftEndStopStCtrl/4(EotDetd)
  [EotDi] -> SoftEndStopStCtrl/3(EotDi)
  [HwAuthy] -> SoftEndStopStCtrl/2(HwAuthy)
  [VehSpd] -> SoftEndStopStCtrl/1(VehSpd)
  Constant5/1 -> If Action Subsystem5/1(In1)

== system SF018A_EotProtn/call_EotProtnInit1/CopyRight2 ==

== system SF018A_EotProtn/EotProtn/EotProtnInit1/CopyRight2 ==

== system SF018A_EotProtn/EotProtn/EotProtnPer1/CopyRight2 ==

== system SF018A_EotProtn/EotProtn/EotProtnPer1/EotDetd ==
  note: Eot management involves one approach at a time.  The system may use the EotVelImpct algorithm or the Soft End Stop algorithm... but never both at the same time.
      | This EotDetd subroutine decides when to switch from original to soft stop.
      |
      | There are three possible reasons to keep using the original algorithm:
      | 1.  Clockwise end of travel has not been found.
      | 2.  Counterclockwise end of travel has not been found.
      | 3.  The soft stop algorithm has been calibrated Off.
  CwDetd : Inport
  CcwDetd : Inport  Port=2
  Constant : Constant  RequirementInfo={'linktype_rmi_doors' '0000ba56 (/E-STEER Core/SubSystem Specifications/Application Functions/SF018A End-of-Travel Actuator Management- EOT Impact and Soft Stops)' '#SF018A_101' 'true' 'REQ: SF018A_101' '' ; 'linktype_rmi_doors' '0000ba56 (/E-STEER Core/SubSystem Specifications/Application Functions/SF018A End-of-Travel Actuator Management- EOT Impact and Soft Stops)' '#SF018A_102' 'true' 'REQ: SF018A_102' '' } %GIDa_882555e4_9e8a_4304_8d5f_b9b17090494c  Value=EotProtnSoftEndStopEna
  CopyRight2 : Subsystem  Description=|  mask(Copyright Information){none=on}
      | Copyright info block.                                               
      |                                                                     
      | Place copyright information at the top of every subsystem in design.
      mask prompts: none "No parameters"
      mask help: Place copyright information at the top of every subsystem in design.
      mask Display:
      | NxtrConf = 'Nexteer Confidential';
      | 
      | sys = bdroot; %handle for the current model ("system")
      | first = get_param(sys,'Created');
      | if(isempty(first))
      |     first = datestr(now,'yyyy');
      | else
      |     first = first(end-3:end);  %year is last four digits
      | end
      | 
      | last = get_param(sys,'LastModifiedDate');
      | if isempty(last)
      |     last = datestr(now,'yyyy');
      | else
      |     last = last(end-3:end);
      | end
      | 
      | if strcmp(first,last)
      |     fprintf('%s -- Copyright %s Nexteer',NxtrConf,first)
      | else
      |     fprintf('%s -- %s%s- %s Nexteer',NxtrConf,char(169),first,last)
      | end
  Data Store Write1 : DataStoreWrite  DataStoreName=dEotProtnDetd
  Logical Operator : Logic  RequirementInfo={'linktype_rmi_doors' '0000ba56 (/E-STEER Core/SubSystem Specifications/Application Functions/SF018A End-of-Travel Actuator Management- EOT Impact and Soft Stops)' '#SF018A_101' 'true' 'REQ: SF018A_101' '' ; 'linktype_rmi_doors' '0000ba56 (/E-STEER Core/SubSystem Specifications/Application Functions/SF018A End-of-Travel Actuator Management- EOT Impact and Soft Stops)' '#SF018A_102' 'true' 'REQ: SF018A_102' '' } %GIDa_743d429d_f6fa_42e6_b920_bdaaa36b9622  Inputs=3  AllPortsSameDT=off  OutDataTypeStr=boolean
  EotDetd : Outport
  wires:
  Logical Operator/1 -> Data Store Write1/1, EotDetd/1
  Constant/1 -> Logical Operator/3
  CcwDetd/1 -> Logical Operator/2
  CwDetd/1 -> Logical Operator/1
